simulink model "untitled"  (R2018a)
settings: Solver=VariableStepAuto  StartTime=0.0  StopTime=20  RelTol=1e-3
undefined symbols (not defined in the file or in its folder): X, Y, Z
libraries: sm_lib x106, nesl_utility x28, simulink x12
(part 2 of 2)

== matlab function untitled/MATLAB Function1 ==
  data: x input; q1 output; y input; z input; q2 output; q3 output
function [q1,q2,q3] = fcn(x,y,z)
L1=1.8;
L2=0.8;
L3=0.4;

q1=atan2(y,x);
q2 = 2*atan((2*L2*(z - L1) - (L2^2*((- L2^2 + 2*L2*L3 - L3^2 + (x/cos((atan2(y,x))))^2 + (z - L1)^2)*(L2^2 + 2*L2*L3 + L3^2 - (x/cos((atan2(y,x))))^2 - (z - L1)^2))^(1/2))/(- L2^2 + 2*L2*L3 - L3^2 + (x/cos((atan2(y,x))))^2 + (z - L1)^2) - (L3^2*((- L2^2 + 2*L2*L3 - L3^2 + (x/cos((atan2(y,x))))^2 + (z - L1)^2)*(L2^2 + 2*L2*L3 + L3^2 - (x/cos((atan2(y,x))))^2 - (z - L1)^2))^(1/2))/(- L2^2 + 2*L2*L3 - L3^2 + (x/cos((atan2(y,x))))^2 + (z - L1)^2) + ((x/cos((atan2(y,x))))^2*((- L2^2 + 2*L2*L3 - L3^2 + (x/cos((atan2(y,x))))^2 + (z - L1)^2)*(L2^2 + 2*L2*L3 + L3^2 - (x/cos((atan2(y,x))))^2 - (z - L1)^2))^(1/2))/(- L2^2 + 2*L2*L3 - L3^2 + (x/cos((atan2(y,x))))^2 + (z - L1)^2) + ((z - L1)^2*((- L2^2 + 2*L2*L3 - L3^2 + (x/cos((atan2(y,x))))^2 + (z - L1)^2)*(L2^2 + 2*L2*L3 + L3^2 - (x/cos((atan2(y,x))))^2 - (z - L1)^2))^(1/2))/(- L2^2 + 2*L2*L3 - L3^2 + (x/cos((atan2(y,x))))^2 + (z - L1)^2) + (2*L2*L3*((- L2^2 + 2*L2*L3 - L3^2 + (x/cos((atan2(y,x))))^2 + (z - L1)^2)*(L2^2 + 2*L2*L3 + L3^2 - (x/cos((atan2(y,x))))^2 - (z - L1)^2))^(1/2))/(- L2^2 + 2*L2*L3 - L3^2 + (x/cos((atan2(y,x))))^2 + (z - L1)^2))/(L2^2 + 2*L2*(x/cos((atan2(y,x)))) - L3^2 + (x/cos((atan2(y,x))))^2 + (z - L1)^2));
q3 = -2*atan(((- L2^2 + 2*L2*L3 - L3^2 + (x/cos((atan2(y,x))))^2 + (z - L1)^2)*(L2^2 + 2*L2*L3 + L3^2 - (x/cos((atan2(y,x))))^2 - (z - L1)^2))^(1/2)/(- L2^2 + 2*L2*L3 - L3^2 + (x/cos((atan2(y,x))))^2 + (z - L1)^2));
end

== matlab function untitled/MATLAB Function ==
  data: x input; q1 output; y input; z input; q2 output; q3 output
function [q1,q2,q3] = fcn(x,y,z)
L1=1.2;
L2=0.8;
L3=0.4;

q1=atan2(y,x);
q2 = 2*atan((2*L2*(z - L1) - (L2^2*((- L2^2 + 2*L2*L3 - L3^2 + (x/cos((atan2(y,x))))^2 + (z - L1)^2)*(L2^2 + 2*L2*L3 + L3^2 - (x/cos((atan2(y,x))))^2 - (z - L1)^2))^(1/2))/(- L2^2 + 2*L2*L3 - L3^2 + (x/cos((atan2(y,x))))^2 + (z - L1)^2) - (L3^2*((- L2^2 + 2*L2*L3 - L3^2 + (x/cos((atan2(y,x))))^2 + (z - L1)^2)*(L2^2 + 2*L2*L3 + L3^2 - (x/cos((atan2(y,x))))^2 - (z - L1)^2))^(1/2))/(- L2^2 + 2*L2*L3 - L3^2 + (x/cos((atan2(y,x))))^2 + (z - L1)^2) + ((x/cos((atan2(y,x))))^2*((- L2^2 + 2*L2*L3 - L3^2 + (x/cos((atan2(y,x))))^2 + (z - L1)^2)*(L2^2 + 2*L2*L3 + L3^2 - (x/cos((atan2(y,x))))^2 - (z - L1)^2))^(1/2))/(- L2^2 + 2*L2*L3 - L3^2 + (x/cos((atan2(y,x))))^2 + (z - L1)^2) + ((z - L1)^2*((- L2^2 + 2*L2*L3 - L3^2 + (x/cos((atan2(y,x))))^2 + (z - L1)^2)*(L2^2 + 2*L2*L3 + L3^2 - (x/cos((atan2(y,x))))^2 - (z - L1)^2))^(1/2))/(- L2^2 + 2*L2*L3 - L3^2 + (x/cos((atan2(y,x))))^2 + (z - L1)^2) + (2*L2*L3*((- L2^2 + 2*L2*L3 - L3^2 + (x/cos((atan2(y,x))))^2 + (z - L1)^2)*(L2^2 + 2*L2*L3 + L3^2 - (x/cos((atan2(y,x))))^2 - (z - L1)^2))^(1/2))/(- L2^2 + 2*L2*L3 - L3^2 + (x/cos((atan2(y,x))))^2 + (z - L1)^2))/(L2^2 + 2*L2*(x/cos((atan2(y,x)))) - L3^2 + (x/cos((atan2(y,x))))^2 + (z - L1)^2));
q3 = -2*atan(((- L2^2 + 2*L2*L3 - L3^2 + (x/cos((atan2(y,x))))^2 + (z - L1)^2)*(L2^2 + 2*L2*L3 + L3^2 - (x/cos((atan2(y,x))))^2 - (z - L1)^2))^(1/2)/(- L2^2 + 2*L2*L3 - L3^2 + (x/cos((atan2(y,x))))^2 + (z - L1)^2));
end

== matlab function untitled/MATLAB Function2 ==
  data: x input; q1 output; y input; z input; q2 output; q3 output
function [q1,q2,q3] = fcn(x,y,z)
L1=0.6;
L2=0.8;
L3=0.4;

q1=atan2(y,x);
q2 = 2*atan((2*L2*(z - L1) - (L2^2*((- L2^2 + 2*L2*L3 - L3^2 + (x/cos((atan2(y,x))))^2 + (z - L1)^2)*(L2^2 + 2*L2*L3 + L3^2 - (x/cos((atan2(y,x))))^2 - (z - L1)^2))^(1/2))/(- L2^2 + 2*L2*L3 - L3^2 + (x/cos((atan2(y,x))))^2 + (z - L1)^2) - (L3^2*((- L2^2 + 2*L2*L3 - L3^2 + (x/cos((atan2(y,x))))^2 + (z - L1)^2)*(L2^2 + 2*L2*L3 + L3^2 - (x/cos((atan2(y,x))))^2 - (z - L1)^2))^(1/2))/(- L2^2 + 2*L2*L3 - L3^2 + (x/cos((atan2(y,x))))^2 + (z - L1)^2) + ((x/cos((atan2(y,x))))^2*((- L2^2 + 2*L2*L3 - L3^2 + (x/cos((atan2(y,x))))^2 + (z - L1)^2)*(L2^2 + 2*L2*L3 + L3^2 - (x/cos((atan2(y,x))))^2 - (z - L1)^2))^(1/2))/(- L2^2 + 2*L2*L3 - L3^2 + (x/cos((atan2(y,x))))^2 + (z - L1)^2) + ((z - L1)^2*((- L2^2 + 2*L2*L3 - L3^2 + (x/cos((atan2(y,x))))^2 + (z - L1)^2)*(L2^2 + 2*L2*L3 + L3^2 - (x/cos((atan2(y,x))))^2 - (z - L1)^2))^(1/2))/(- L2^2 + 2*L2*L3 - L3^2 + (x/cos((atan2(y,x))))^2 + (z - L1)^2) + (2*L2*L3*((- L2^2 + 2*L2*L3 - L3^2 + (x/cos((atan2(y,x))))^2 + (z - L1)^2)*(L2^2 + 2*L2*L3 + L3^2 - (x/cos((atan2(y,x))))^2 - (z - L1)^2))^(1/2))/(- L2^2 + 2*L2*L3 - L3^2 + (x/cos((atan2(y,x))))^2 + (z - L1)^2))/(L2^2 + 2*L2*(x/cos((atan2(y,x)))) - L3^2 + (x/cos((atan2(y,x))))^2 + (z - L1)^2));
q3 = -2*atan(((- L2^2 + 2*L2*L3 - L3^2 + (x/cos((atan2(y,x))))^2 + (z - L1)^2)*(L2^2 + 2*L2*L3 + L3^2 - (x/cos((atan2(y,x))))^2 - (z - L1)^2))^(1/2)/(- L2^2 + 2*L2*L3 - L3^2 + (x/cos((atan2(y,x))))^2 + (z - L1)^2));
end

== matlab function untitled/MATLAB Function3 ==
  data: x output; t input; y output; z output
function [x,y,z] = fcn(t)

if (t<5.0)
    x = -0.18*t + 1.2;
    y = 0.1*t;
    z = 1.2;
elseif (t<10.0)
    x=0.3;
    y=0.5;
    z=1.2;
elseif (t<15.0)
    x = 0.18*t - 1.5;
    y = -0.1*t + 1.5;
    z = 1.2;
else
    x=1.2;
    y=0.0;
    z=1.2;
end
  
end

== matlab function untitled/MATLAB Function4 ==
  data: x output; t input; y output; z output
function [x,y,z] = fcn(t)

if (t<5.0)
    x = -0.18*t + 1.2;
    y = 0.1*t;
    z = -0.12*t + 1.8;
elseif (t<15.0)
    x=0.3;
    y=0.5;
    z=1.2;
else
   x = 0.18*t - 2.4;
   y = -0.1*t + 2.0;
   z = 0.12*t - 0.6;
end
  
end

== matlab function untitled/MATLAB Function5 ==
  data: x output; t input; y output; z output
function [x,y,z] = fcn(t)

if (t<5.0)
    x = -0.18*t + 1.2;
    y = 0.1*t;
    z = 0.12*t + 0.6;
elseif (t<10.0)
    x = 0.18*t - 0.6;
    y = -0.1*t + 1.0;
    z = -0.12*t + 1.8;
else
    x=1.2;
    y=0.0;
    z=0.6;
end
  
end
